simulink model "NonlinearHinf"  (R2019a)
settings: Solver=VariableStepAuto  StartTime=0.0  StopTime=10  FixedStep=0.002  RelTol=1e-3  EnableMultiTasking=on
libraries: cstblocks x1, simulink_extras x1
settings Model: ExtModeTrigDuration=10000  Creator=marcos.pesante  LastModifiedBy=marcos.pesante
settings SolverCC: PositivePriorityOrder=on
settings RTWCC: SystemTargetFile=quarc_win64.tlc  TemplateMakefile=quarc_default_tmf  Description=QUARC Win64 Target
settings STFCustomTargetCC: TargetPreCompLibLocation=C:\PROGRA~3\QUARC\lib\2019a\win64\release  TargetLangStandard=C99 (ISO)  ConcurrentExecutionCompliant=on  SystemTargetFile=quarc_win64.tlc
settings GRTTargetCC: TargetPreCompLibLocation=C:\PROGRA~3\QUARC\lib\2019a\win64\release  ParMdlRefBuildCompliant=off  CompOptLevelCompliant=off  CombineOutputUpdateFcns=off  MatFileLogging=off  CPPClassGenCompliant=off  GRTInterface=on  UseToolchainInfoCompliant=off  ExtMode=on  ExtModeMexFile=quarc_comm

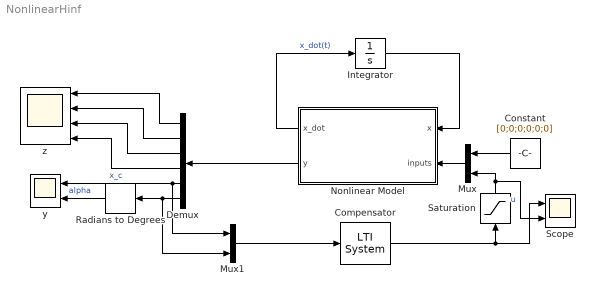
== system NonlinearHinf ==
  Compensator : cstblocks/LTI System  sys=K  IC=[]
  Constant : Constant  Value=[0;0;0;0;0;0]
  Demux : Demux  Outputs=6
  Integrator : Integrator  InitialCondition=[0;3 * pi / 180;0;0]
  Mux : Mux  Inputs=2
  Mux1 : Mux  Inputs=2
  Nonlinear Model : MATLAB Function  TreatAsAtomicUnit=on
  Radians to Degrees : simulink_extras/Transformations/Radians to Degrees
  Saturation : Saturate  UpperLimit=5  LowerLimit=-5  OutDataTypeStr=double
  Scope : Scope  NumInputPorts=2
  y : Scope  NumInputPorts=2
  z : Scope  NumInputPorts=4
  wires:
  Demux/3 -> z/3
  Demux/1 -> z/1
  Demux/2 -> z/2
  Mux1/1 -> Compensator/1
  Demux/4 -> z/4
  Radians to Degrees/1 -> y/2  "alpha"
  Mux/1 -> Nonlinear Model/2(inputs)
  Constant/1 -> Mux/1
  Demux/6 -> Mux1/2, Radians to Degrees/1
  Demux/5 -> y/1, Mux1/1  "x_c"
  Nonlinear Model/2(y) -> Demux/1
  Nonlinear Model/1(x_dot) -> Integrator/1  "x_dot(t)"
  Integrator/1 -> Nonlinear Model/1(x)
  Saturation/1 -> Mux/2, Scope/2  "u"
  Compensator/1 -> Scope/1, Saturation/1

== matlab function NonlinearHinf/Nonlinear Model ==
  data: x_dot output size=4; x input size=4; inputs input; y output
function [x_dot, y] = NonlinearModel(x, inputs)
    x_c = x(1);
    alpha = x(2);
    x_c_dot = x(3);
    alpha_dot = x(4);
    
    x_ref = inputs(1);
    x_dot_ref = inputs(2);
    alpha_ref = inputs(3);
    alpha_dot_ref = inputs(4);
    F_d = inputs(5);
    Tau_d = inputs(6);
    V_m = inputs(7);
    
    x_dot = [
        x_c_dot;
        alpha_dot;
        (0.035320935178499876438522107813446*V_m)/(0.005767794916*sin(alpha)^2 + 0.030917930772731869127468717906027) - (0.0329573692*F_d)/(0.005767794916*sin(alpha)^2 + 0.030917930772731869127468717906027) - (0.35623119816912776053346814385936*x_c_dot)/(0.005767794916*sin(alpha)^2 + 0.030917930772731869127468717906027) - (0.0025029803612632*alpha_dot^2*sin(alpha))/(0.005767794916*sin(alpha)^2 + 0.030917930772731869127468717906027) + (0.05658206812596*cos(alpha)*sin(alpha))/(0.005767794916*sin(alpha)^2 + 0.030917930772731869127468717906027) - (0.075946*Tau_d*cos(alpha))/(0.005767794916*sin(alpha)^2 + 0.030917930772731869127468717906027) - (0.0037973*alpha_dot*cos(alpha))/(0.005767794916*sin(alpha)^2 + 0.030917930772731869127468717906027);
        (0.82931303109486613774754788508403*sin(alpha))/(0.005767794916*sin(alpha)^2 + 0.030917930772731869127468717906027) - (1.11312664145328290121739200913*Tau_d)/(0.005767794916*sin(alpha)^2 + 0.030917930772731869127468717906027) - (0.055656332072664145060869600456499*alpha_dot)/(0.005767794916*sin(alpha)^2 + 0.030917930772731869127468717906027) - (0.075946*F_d*cos(alpha))/(0.005767794916*sin(alpha)^2 + 0.030917930772731869127468717906027) + (0.08139253248*V_m*cos(alpha))/(0.005767794916*sin(alpha)^2 + 0.030917930772731869127468717906027) - (0.82088877944033763779527559055118*x_c_dot*cos(alpha))/(0.005767794916*sin(alpha)^2 + 0.030917930772731869127468717906027) - (0.005767794916*alpha_dot^2*cos(alpha)*sin(alpha))/(0.005767794916*sin(alpha)^2 + 0.030917930772731869127468717906027);
    ];

    y = [
        x_ref - x_c;
        x_dot_ref - x_c_dot;
        alpha_ref - alpha;
        alpha_dot_ref - alpha_dot;
        x_c;
        alpha
    ];
